simulink library "lib_Convection_CylCrossFlowHilpert"  (R2015a)
settings: Solver=ode45  StartTime=0.0  StopTime=10.0  RelTol=1e-3
libraries: simulink x11, lib_GenTools_MinMax x1
settings Model: Creator=jlkratz  LastModifiedBy=jlkratz

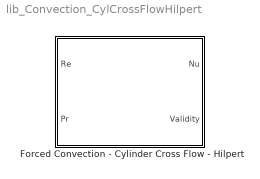
== system lib_Convection_CylCrossFlowHilpert ==
  Forced Convection - Cylinder Cross Flow - Hilpert : Subsystem  mask(TSAT: Cylinder Cross Flow - Hilpert){}
      mask help:
      | This block estimates the average Nusselt number of an external flow over an isothermal cylinder. The correlation employed was originally developed by Hilpert and has been modified to account for fluids with a wider range of Prandtl numbers. Note that all fluid properrties should be evaluated at film temperature (average of the bulk fluid and surface temperatures). Also the Reynolds number uses the diameter of the cylinder as the characteristic length. The correlation is subject to the following restrictions:
      |
      | 1 <= Re <= 1000000
      | 0.7 <= Pr <= 500
      |
      | For more information see the block help menu.
      mask Help: web(which('Convection_TSAT_CylinderCrossFlowHilpert.html'),'-helpbrowser')

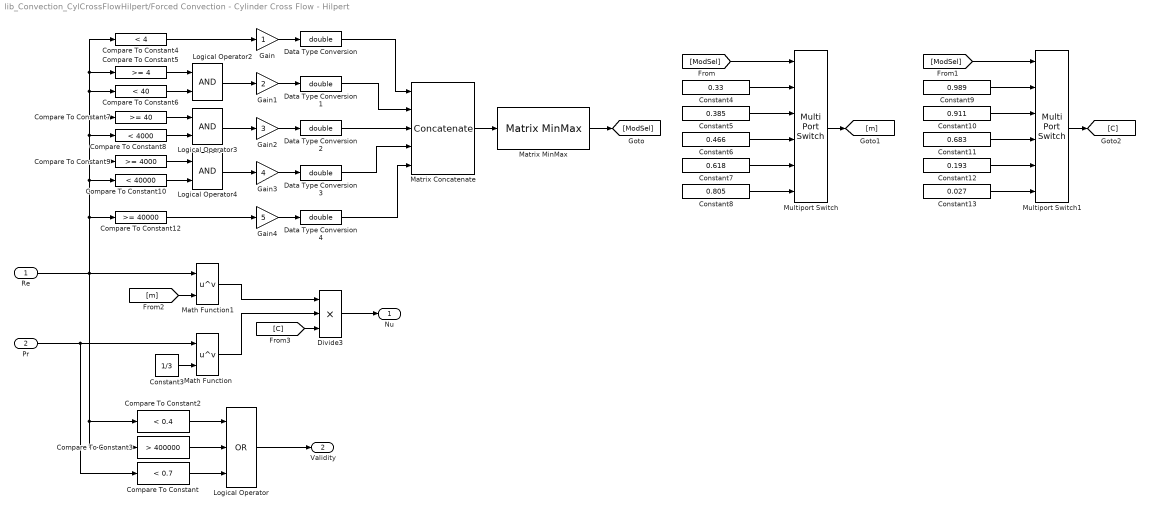
== system lib_Convection_CylCrossFlowHilpert/Forced Convection - Cylinder Cross Flow - Hilpert ==
  Re : Inport
  Pr : Inport  Port=2
  Compare To Constant : simulink/Logic and Bit Operations/Compare To Constant  relop=<  const=0.7  OutDataTypeStr=boolean
  Compare To Constant10 : simulink/Logic and Bit Operations/Compare To Constant  relop=<  const=40000  OutDataTypeStr=boolean
  Compare To Constant12 : simulink/Logic and Bit Operations/Compare To Constant  relop=>=  const=40000  OutDataTypeStr=boolean
  Compare To Constant2 : simulink/Logic and Bit Operations/Compare To Constant  relop=<  const=0.4  OutDataTypeStr=boolean
  Compare To Constant3 : simulink/Logic and Bit Operations/Compare To Constant  relop=>  const=400000  OutDataTypeStr=boolean
  Compare To Constant4 : simulink/Logic and Bit Operations/Compare To Constant  relop=<  const=4  OutDataTypeStr=boolean
  Compare To Constant5 : simulink/Logic and Bit Operations/Compare To Constant  relop=>=  const=4  OutDataTypeStr=boolean
  Compare To Constant6 : simulink/Logic and Bit Operations/Compare To Constant  relop=<  const=40  OutDataTypeStr=boolean
  Compare To Constant7 : simulink/Logic and Bit Operations/Compare To Constant  relop=>=  const=40  OutDataTypeStr=boolean
  Compare To Constant8 : simulink/Logic and Bit Operations/Compare To Constant  relop=<  const=4000  OutDataTypeStr=boolean
  Compare To Constant9 : simulink/Logic and Bit Operations/Compare To Constant  relop=>=  const=4000  OutDataTypeStr=boolean
  Constant10 : Constant  Value=0.911
  Constant11 : Constant  Value=0.683
  Constant12 : Constant  Value=0.193
  Constant13 : Constant  Value=0.027
  Constant3 : Constant  Value=1/3
  Constant4 : Constant  Value=0.33
  Constant5 : Constant  Value=0.385
  Constant6 : Constant  Value=0.466
  Constant7 : Constant  Value=0.618
  Constant8 : Constant  Value=0.805
  Constant9 : Constant  Value=0.989
  Data Type Conversion{,1..4} (5 alike) : DataTypeConversion  OutDataTypeStr=double
  Divide3 : Product  Inputs=***
  Gain : Gain
  Gain1 : Gain  Gain=2
  Gain2 : Gain  Gain=3
  Gain3 : Gain  Gain=4
  Gain4 : Gain  Gain=5
  Logical Operator : Logic  Operator=OR  Inputs=3  AllPortsSameDT=off  OutDataTypeStr=boolean
  Logical Operator2 : Logic  AllPortsSameDT=off  OutDataTypeStr=boolean
  Logical Operator3 : Logic  AllPortsSameDT=off  OutDataTypeStr=boolean
  Logical Operator4 : Logic  AllPortsSameDT=off  OutDataTypeStr=boolean
  Math Function : Math  Operator=pow  SaturateOnIntegerOverflow=on
  Math Function1 : Math  Operator=pow  SaturateOnIntegerOverflow=on
  Matrix Concatenate : Concatenate  NumInputs=5  Mode=Multidimensional array  ConcatenateDimension=2
  Matrix MinMax : lib_GenTools_MinMax/Matrix MinMax  rows_M=on  cols_M=off  all_M=off  minmax_M=off  BN_M=gcb
  Multiport Switch : MultiPortSwitch  Inputs=5
  Multiport Switch1 : MultiPortSwitch  Inputs=5
  Nu : Outport
  Validity : Outport  Port=2
  wires:
  Matrix Concatenate/1 -> Matrix MinMax/1
  Data Type Conversion4/1 -> Matrix Concatenate/5
  Data Type Conversion3/1 -> Matrix Concatenate/4
  Data Type Conversion2/1 -> Matrix Concatenate/3
  Data Type Conversion1/1 -> Matrix Concatenate/2
  Data Type Conversion/1 -> Matrix Concatenate/1
  Matrix MinMax/1 -> [ModSel]
  Divide3/1 -> Nu/1
  [C] -> Divide3/3
  Constant13/1 -> Multiport Switch1/6
  Constant12/1 -> Multiport Switch1/5
  Constant11/1 -> Multiport Switch1/4
  Constant10/1 -> Multiport Switch1/3
  Constant9/1 -> Multiport Switch1/2
  Constant8/1 -> Multiport Switch/6
  Constant7/1 -> Multiport Switch/5
  Constant6/1 -> Multiport Switch/4
  Constant5/1 -> Multiport Switch/3
  Constant4/1 -> Multiport Switch/2
  Multiport Switch1/1 -> [C]
  Multiport Switch/1 -> [m]
  [ModSel] -> Multiport Switch1/1
  [ModSel] -> Multiport Switch/1
  Compare To Constant4/1 -> Gain/1
  Logical Operator2/1 -> Gain1/1
  Logical Operator3/1 -> Gain2/1
  Logical Operator4/1 -> Gain3/1
  Compare To Constant12/1 -> Gain4/1
  Gain4/1 -> Data Type Conversion4/1
  Gain3/1 -> Data Type Conversion3/1
  Gain2/1 -> Data Type Conversion2/1
  Gain1/1 -> Data Type Conversion1/1
  Gain/1 -> Data Type Conversion/1
  Compare To Constant9/1 -> Logical Operator4/1
  Compare To Constant10/1 -> Logical Operator4/2
  Compare To Constant7/1 -> Logical Operator3/1
  Compare To Constant8/1 -> Logical Operator3/2
  Compare To Constant5/1 -> Logical Operator2/1
  Compare To Constant6/1 -> Logical Operator2/2
  Logical Operator/1 -> Validity/1
  Compare To Constant/1 -> Logical Operator/3
  Compare To Constant3/1 -> Logical Operator/2
  Compare To Constant2/1 -> Logical Operator/1
  Math Function/1 -> Divide3/2
  Math Function1/1 -> Divide3/1
  [m] -> Math Function1/2
  Constant3/1 -> Math Function/2
  Pr/1 -> Compare To Constant/1, Math Function/1
  Re/1 -> Math Function1/1, Compare To Constant3/1, Compare To Constant2/1, Compare To Constant12/1, Compare To Constant4/1, Compare To Constant5/1, Compare To Constant6/1, Compare To Constant7/1, Compare To Constant8/1, Compare To Constant9/1, Compare To Constant10/1
